simulink model "final_quadruped_200622"  (R2021a)
settings: Solver=ode15s  StartTime=0.0  StopTime=10  FixedStep=1e-3  RelTol=1e-5  EnableMultiTasking=on
values from neighbouring files (symbols this model uses):
  foot_x = 8    [bipedparameters.m]    (also in fcn.m; finalrobotParameters.m; finalrobotParameters_110522.m; finalrobotParameters_140522.m)
  foot_y = 6    [bipedparameters.m]    (also in fcn.m; finalrobotParameters.m; finalrobotParameters_110522.m; finalrobotParameters_140522.m)
  foot_z = 1    [bipedparameters.m]    (also in fcn.m; finalrobotParameters.m; finalrobotParameters_110522.m; finalrobotParameters_140522.m)
  height_plane = 0.025    [bipedparameters.m]    (also in finalrobotParameters.m; finalrobotParameters_110522.m; finalrobotParameters_140522.m; finalrobotParameters_240522.m)
  kd_ankle = 1000    [bipedparameters.m]    (also in finalrobotParameters_240522.m)
  kd_hip = 1000    [bipedparameters.m]    (also in finalrobotParameters_240522.m)
  kd_knee = 1000    [bipedparameters.m]    (also in finalrobotParameters_240522.m)
  ki_ankle = 1000    [bipedparameters.m]    (also in finalrobotParameters_240522.m)
  ki_hip = 1000    [bipedparameters.m]    (also in finalrobotParameters_240522.m)
  ki_knee = 2000    [bipedparameters.m]    (also in finalrobotParameters_240522.m)
  kp_ankle = 1000    [bipedparameters.m]    (also in finalrobotParameters_240522.m)
  kp_hip = 1000    [bipedparameters.m]    (also in finalrobotParameters_240522.m)
  kp_knee = 2000    [bipedparameters.m]    (also in finalrobotParameters_240522.m)
  lower_leg_length = 10    [bipedparameters.m]    (also in fcn.m; finalrobotParameters.m; finalrobotParameters_110522.m; finalrobotParameters_140522.m)
  m_ll = density*leg_radius*leg_radius*lower_leg_length*3.141592653589*0.01*0.01*0.01    (= 0.0176714586764)    [bipedparameters.m]    (also in fcn.m; finalrobotParameters_140522.m; finalrobotParameters_240522.m; hdotlb.m)
  m_ul = density*leg_radius*leg_radius*upper_leg_length*3.141592653589*0.01*0.01*0.01    (= 0.0176714586764)    [bipedparameters.m]    (also in fcn.m; finalrobotParameters_140522.m; finalrobotParameters_240522.m; hdotlb.m)
  plane_x = 25    [bipedparameters.m]    (also in finalrobotParameters.m; finalrobotParameters_110522.m; finalrobotParameters_140522.m; finalrobotParameters_240522.m)
  plane_y = 3    [bipedparameters.m]    (also in finalrobotParameters.m; finalrobotParameters_110522.m; finalrobotParameters_140522.m; finalrobotParameters_240522.m)
  torso_offset_x = -0.5    [bipedparameters.m]    (also in finalrobotParameters.m = 10; finalrobotParameters_110522.m = 10; finalrobotParameters_140522.m = 10; finalrobotParameters_240522.m = 10)
  torso_offset_z = -2    [bipedparameters.m]    (also in finalrobotParameters.m; finalrobotParameters_110522.m; finalrobotParameters_140522.m; finalrobotParameters_240522.m)
  torso_x = 5    [bipedparameters.m]    (also in fcn.m = 25; finalrobotParameters.m = 25; finalrobotParameters_110522.m = 25; finalrobotParameters_140522.m = 25)
  torso_y = 10    [bipedparameters.m]    (also in fcn.m = 16; finalrobotParameters.m = 16; finalrobotParameters_110522.m = 16; finalrobotParameters_140522.m = 16)
  torso_z = 8    [bipedparameters.m]    (also in fcn.m = 10; finalrobotParameters.m = 10; finalrobotParameters_110522.m = 10; finalrobotParameters_140522.m = 10)
  upper_leg_length = 10    [bipedparameters.m]    (also in fcn.m; finalrobotParameters.m; finalrobotParameters_110522.m; finalrobotParameters_140522.m)
undefined symbols (not defined in the file or in its folder): sigbuilder_block, X, Y, Z
libraries: nesl_utility x188, sm_lib x71, Contact_Forces_Lib x16, pid_lib x12, fl_lib x3
(part 8 of 8)

== matlab function final_quadruped_200622/Subsystem/MATLAB Function3 ==
  data: px input; py input; pz input; p output; vx input; vy input; v output; vz input; ax input; ay input; az input; a output
function [p,v,a] = fcn(px,py,pz,vx,vy,vz,ax,ay,az)
p=[px;py;pz];
v=[vx;vy;vz];
a=[ax;ay;az];
end

== matlab function final_quadruped_200622/Model/Left LegBack/MATLAB Function1 ==
  data: ankle input; knee input; t2dLB output; hip input
function t2dLB= fcn(ankle, knee, hip)
t2dLB=[hip;knee;ankle];
end

== matlab function final_quadruped_200622/Subsystem/MATLAB Function ==
  data: aulRF input; Macm output; allRF input; afRF input; aulLF input; allLF input; afLF input; aulRB input; allRB input; afRB input; aulLB input; allLB input; afLB input; a_torso input; alinks output; acm output
function [Macm,alinks,acm] = fcn(aulRF,allRF,afRF,aulLF,allLF,afLF,aulRB,allRB,afRB,aulLB,allLB,afLB,a_torso)
%%
lower_leg_length = 10;
upper_leg_length = 10;
density = 1000;
foot_density=2000;
leg_radius = 0.75;
foot_x = 8;
foot_y = 6;
foot_z = 1;
torso_y = 16;
torso_x = 25;
torso_z = 10;
m_ul=density*leg_radius*leg_radius*upper_leg_length*3.141592653589*0.01*0.01*0.01;
m_ll=density*leg_radius*leg_radius*lower_leg_length*3.141592653589*0.01*0.01*0.01;
m_foot=foot_density*foot_x*foot_y*foot_z*0.000001;
m_torso=density*torso_x*torso_y*torso_z*0.000001;
M=m_torso+4*(m_ul+m_ll+m_foot);
%%
Macm=m_torso*a_torso+(m_ul*aulRF+m_ll*allRF+m_foot*afRF)+(m_ul*aulLF+m_ll*allLF+m_foot*afLF)+(m_ul*aulRB+m_ll*allRB+m_foot*afRB)+(m_ul*aulLB+m_ll*allLB+m_foot*afLB);
alinks=[aulRF allRF afRF aulLF allLF afLF aulRB allRB afRB aulLB allLB afLB];
acm=Macm/M;
end

== matlab function final_quadruped_200622/Subsystem/MATLAB Function15 ==
  data: pulRF input; pllRF input; pfRF input; pulLF input; pllLF input; pfLF input; pulRB input; pllRB input; pfRB input; pulLB input; pllLB input; pfLB input; p_torso input; pcm output
function pcm = fcn(pulRF,pllRF,pfRF,pulLF,pllLF,pfLF,pulRB,pllRB,pfRB,pulLB,pllLB,pfLB,p_torso)
%%
lower_leg_length = 10;
upper_leg_length = 10;
density = 1000;
foot_density=2000;
leg_radius = 0.75;
foot_x = 8;
foot_y = 6;
foot_z = 1;
torso_y = 16;
torso_x = 25;
torso_z = 10;
m_ul=density*leg_radius*leg_radius*upper_leg_length*3.141592653589*0.01*0.01*0.01;
m_ll=density*leg_radius*leg_radius*lower_leg_length*3.141592653589*0.01*0.01*0.01;
m_foot=foot_density*foot_x*foot_y*foot_z*0.000001;
m_torso=density*torso_x*torso_y*torso_z*0.000001;
M=m_torso+4*(m_ul+m_ll+m_foot);
%%
Mpcm=m_torso*p_torso+(m_ul*pulRF+m_ll*pllRF+m_foot*pfRF)+(m_ul*pulLF+m_ll*pllLF+m_foot*pfLF)+(m_ul*pulRB+m_ll*pllRB+m_foot*pfRB)+(m_ul*pulLB+m_ll*pllLB+m_foot*pfLB);
plinks=[pulRF pllRF pfRF pulLF pllLF pfLF pulRB pllRB pfRB pulLB pllLB pfLB];
pcm=Mpcm/M;
end
